simulink library "mach_lib"  (Simulink 6.3)
undefined symbols (not defined in the file): accel_cmd, aero_surf_qbar_off, aero_surf_qbar_on, altitude_stop, angular_rate_stop, att_cmd_select, att_trim_IC, att_type, att_type_numbers, bb_ellipsoid, bb_params, chi_trim_IC, command_time, compute_all_rate_cols, compute_all_vel_cols, constants, cosA, da_trim_IC, de_trim_IC, DiscIntNeverNeededParam, dr_trim_IC, dtsim, E_rwy, E_trim_IC, Ed_cmd, Ed_trim_IC, energy_stop, eow_boundary, full_surf_llim, full_surf_ulim, gain_var_struct, gam_cmd_descent, gam_cmd_preflare, gamdot_cmd_descent, gamdot_cmd_flare, gamdot_cmd_preflare, gamma_trim_IC, h_trim_IC, hd_cmd, hd_trim_IC, ideal_vel_Kb, integrate_start_time_sim, integrate_state_sim, llim, MACH, MACH_att_fb, MACH_gain_mat, MACH_mass_IC, MACH_pos_IC, MACH_pqr_Bmat_IC, MACH_pqr_IC, MACH_pqr_u_IC, MACH_quat_IC, MACH_throttle_IC, MACH_U_nom_IC, MACH_vel_Bmat_IC, MACH_vel_cvdnom_IC, MACH_vel_IC, MACH_vel_uold_IC, max_chi_cmd ... (+67)
libraries: simulink x75, mach_lib x27, utility_lib x25, model_lib x7, models x6
(part 3 of 6)

== system mach_lib/claw_main/input processing/set control parameters ==
  note: (Optionally) disable bb
      |  while we still have fuel
  signal_bus : Inport
  full_surf : Inport  Port=2
  Bus Creator1 : BusCreator  Inputs=10
  Bus Selector1 : BusSelector  OutputSignals=mode_sw.enable_bb_sw,mode_sw.gain_set_sw
  Bus Selector3 : BusSelector  OutputSignals=aero_env_est
  Constant : Constant
  Constant1 : Constant
  Logical Operator : Logic  Operator=NOT  AllPortsSameDT=off
  Logical Operator1 : Logic  Operator=NOT  AllPortsSameDT=off
  Logical Operator4 : Logic  AllPortsSameDT=off
  Logical Operator5 : Logic  Operator=OR  AllPortsSameDT=off
  accel submode setup : Subsystem
  modify MACH_att_Kf : Subsystem
  out of fuel : model_lib/out of fuel ?
  select gains : Subsystem
  set att desdyn params : Subsystem
  set pos desdyn params : Subsystem
  set rate desdyn params : Subsystem
  set rate di params : Subsystem
  set vel desdyn params : Subsystem
  control_params : Outport
  wires:
  modify MACH_att_Kf/1(gain_bus) -> set att desdyn params/1(gain_bus)
  full_surf/1 -> set rate di params/1(full_surf)
  Bus Selector3/1 -> set rate di params/2(aero_env_est)  "<aero_env_est>"
  set rate di params/1(rate_params) -> Bus Creator1/10  "rate_params"
  signal_bus/1 -> modify MACH_att_Kf/2(signal_bus), Bus Selector3/1, Bus Selector1/1, accel submode setup/1(signal_bus)
  accel submode setup/1(accel_cmd_sw) -> Bus Creator1/1  "accel_cmd_sw"
  accel submode setup/2(accel_cmd) -> Bus Creator1/2  "accel_cmd"
  Bus Selector1/2 -> select gains/2(gain_set_in)  "<gain_set_sw>"
  Constant1/1 -> Logical Operator5/2
  Logical Operator5/1 -> Logical Operator4/2
  Logical Operator1/1 -> Logical Operator5/1
  out of fuel/1 -> Logical Operator1/1
  Constant/1 -> out of fuel/1
  select gains/1(gain_set) -> Bus Creator1/5  "gain_set"
  Bus Creator1/1 -> control_params/1
  select gains/2(gain_bus) -> modify MACH_att_Kf/1(gain_bus_in), set rate desdyn params/1(gain_bus), set vel desdyn params/1(gain_bus), set pos desdyn params/1(gain_bus)
  Logical Operator4/1 -> Bus Creator1/4, Logical Operator/1, select gains/1(enable_bb)  "enable_bb"
  Logical Operator/1 -> Bus Creator1/3  "limit_pqr_cmd"
  Bus Selector1/1 -> Logical Operator4/1  "<enable_bb_sw>"
  set rate desdyn params/1(params) -> Bus Creator1/9  "rate_desdyn"
  set att desdyn params/1(params) -> Bus Creator1/8  "att_desdyn"
  set vel desdyn params/1(params) -> Bus Creator1/7  "vel_desdyn"
  set pos desdyn params/1(params) -> Bus Creator1/6  "pos_desdyn"

== system mach_lib/claw_main/pos_loops/compute trim ==
  inner cmd : Inport
  cmd : Inport  Port=2
  Sum1 : Sum  Inputs=|+-  SaturateOnIntegerOverflow=on
  trim : Outport
  wires:
  cmd/1 -> Sum1/2
  inner cmd/1 -> Sum1/1
  Sum1/1 -> trim/1

== system mach_lib/claw_main/pos_loops/limiter ==
  vel_inner_cmd : Inport
  signal_bus : Inport  Port=2
  cvd_des_in : Inport  Port=3
  Bus Selector2 : BusSelector  OutputSignals=cmd_bus.select_cmd.vel,feed_forward.pos_ff,y_meas.dc_fltpath
  Compare To Constant : simulink/Logic and Bit Operations/Compare To Constant  relop=<  const=2  LogicOutDataTypeMode=boolean  ZeroCross=off
  Constant : Constant  Value=use_pos_fltpath_lim
  Math Function : Math  Operator=transpose  SaturateOnIntegerOverflow=on
  Product : Product  Multiplication=Matrix(*)  RndMeth=Zero
  Product1 : Product  Multiplication=Matrix(*)  RndMeth=Zero
  Saturation : Saturate  UpperLimit=MACH.pos_u_ulim  LowerLimit=MACH.pos_u_llim
  Saturation1 : Saturate  UpperLimit=MACH.pos_fltpath_u_ulim  LowerLimit=MACH.pos_fltpath_u_llim
  Selector1 : Selector  Elements=[1 2 4]  InputPortWidth=4
  Sum : Sum  Inputs=-+|
  Sum1 : Sum  Inputs=++|
  Sum2 : Sum  Inputs=+-|  SaturateOnIntegerOverflow=on  InputSameDT=on
  Switch : Switch  Threshold=0.5
  Switch1 : Switch  Threshold=0.5
  Unit Delay : UnitDelay  X0=MACH_vel_IC  SampleTime=MACH.dt
  cvd_des : Outport
  cvd_extra : Outport  Port=2
  wires:
  vel_inner_cmd/1 -> Unit Delay/1
  Unit Delay/1 -> Switch1/1
  Selector1/1 -> Compare To Constant/1
  Compare To Constant/1 -> Switch1/2
  Bus Selector2/2 -> Switch1/3  "<pos_ff>"
  Bus Selector2/1 -> Selector1/1  "<vel>"
  signal_bus/1 -> Bus Selector2/1
  Sum2/1 -> cvd_extra/1
  Product1/1 -> Sum1/2
  Math Function/1 -> Product1/1
  Saturation1/1 -> Product1/2
  Product/1 -> Saturation1/1
  Sum/1 -> Product/2
  Bus Selector2/3 -> Math Function/1, Product/1  "<dc_fltpath>"
  cvd_des_in/1 -> Sum2/2, Saturation/1, Sum/2
  Sum1/1 -> Switch/1
  Switch/1 -> Sum2/1, cvd_des/1
  Saturation/1 -> Switch/3
  Constant/1 -> Switch/2
  Switch1/1 -> Sum/1, Sum1/1

== system mach_lib/claw_main/pos_loops/select pos cmd ==
  NEh_current : Inport
  outer cmd : Inport  Port=2
  signal_bus : Inport  Port=3
  Bus Selector : BusSelector  OutputSignals=cmd_bus.select_cmd.pos,cmd_bus.autopilot_cmd
  Demux3 : Demux  Outputs=[ 3 1 ]
  Ground : Ground
  Multiport Switch : MultiPortSwitch  Inputs=3  zeroidx=on  SaturateOnIntegerOverflow=on
  Mux1 : Mux  Inputs=2
  Selector2 : Selector  Elements=[1 2 4 3]  InputPortWidth=4
  Selector4 : Selector  Elements=[1 2 4 3]  InputPortWidth=4
  NEh_cmd : Outport
  cam_cmd : Outport  Port=2
  cmd : Outport  Port=3
  wires:
  signal_bus/1 -> Bus Selector/1
  Demux3/2 -> cam_cmd/1
  Demux3/1 -> NEh_cmd/1
  Selector4/1 -> Demux3/1
  Selector2/1 -> Multiport Switch/2
  Mux1/1 -> Selector2/1
  Ground/1 -> Mux1/2
  NEh_current/1 -> Mux1/1
  Bus Selector/1 -> Multiport Switch/1  "<pos>"
  Bus Selector/2 -> Multiport Switch/3  "<autopilot_cmd>"
  outer cmd/1 -> Multiport Switch/4
  Multiport Switch/1 -> Selector4/1, cmd/1

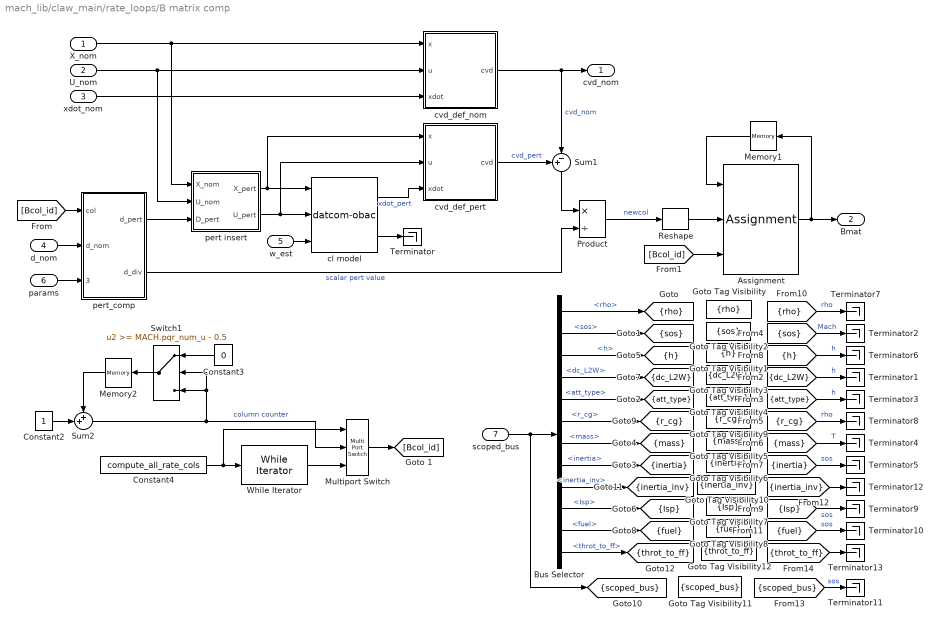
== system mach_lib/claw_main/rate_loops/B matrix comp ==
  X_nom : Inport
  U_nom : Inport  Port=2
  xdot_nom : Inport  Port=3
  d_nom : Inport  Port=4
  w_est : Inport  Port=5
  params : Inport  Port=6
  scoped_bus : Inport  Port=7
  Assignment : Assignment  InputType=Matrix  Rows=-1  ColumnSrc=External
  Bus Selector : BusSelector  OutputSignals=atmos_env.rho,atmos_env.sos,atmos_env.h,dc_L2W,att_type,mass_props.r_cg,mass_props.mass,mass_props.inertia,mass_props.inertia_inv,mass_props.Isp,mass_props.fuel,mass_props.throt_to_ff
  Constant2 : Constant
  Constant3 : Constant  Orientation=left  Value=0
  Constant4 : Constant  Value=compute_all_rate_cols
  Goto Tag Visibility : GotoTagVisibility  GotoTag=rho
  Goto Tag Visibility1 : GotoTagVisibility  GotoTag=h
  Goto Tag Visibility10 : GotoTagVisibility  GotoTag=inertia_inv
  Goto Tag Visibility11 : GotoTagVisibility  GotoTag=scoped_bus
  Goto Tag Visibility12 : GotoTagVisibility  GotoTag=throt_to_ff
  Goto Tag Visibility2 : GotoTagVisibility  GotoTag=sos
  Goto Tag Visibility3 : GotoTagVisibility  GotoTag=dc_L2W
  Goto Tag Visibility4 : GotoTagVisibility  GotoTag=att_type
  Goto Tag Visibility5 : GotoTagVisibility  GotoTag=mass
  Goto Tag Visibility6 : GotoTagVisibility  GotoTag=inertia
  Goto Tag Visibility7 : GotoTagVisibility  GotoTag=Isp
  Goto Tag Visibility8 : GotoTagVisibility  GotoTag=fuel
  Goto Tag Visibility9 : GotoTagVisibility  GotoTag=r_cg
  Memory1 : Memory  Orientation=left  X0=MACH_pqr_Bmat_IC  InheritSampleTime=on
  Memory2 : Memory  Orientation=left  InheritSampleTime=on
  Multiport Switch : MultiPortSwitch  Inputs=2  zeroidx=on
  Product : Product  Inputs=*/  SaturateOnIntegerOverflow=on  InputSameDT=on
  Reshape : simulink/Math Operations/Reshape  OutputDimensionality=Column vector  OutputDimensions=[1,1]
  Sum1 : Sum  Orientation=down  Inputs=+-|  SaturateOnIntegerOverflow=on  InputSameDT=on
  Sum2 : Sum  Inputs=++|  SaturateOnIntegerOverflow=on  InputSameDT=on
  Switch1 : Switch  Orientation=left  Threshold=MACH.pqr_num_u - 0.5  SaturateOnIntegerOverflow=on  InputSameDT=on
  Terminator{,1..13} (14 alike) : Terminator
  While Iterator : WhileIterator  MaxIters=MACH.pqr_num_u  WhileBlockType=do-while  ShowIterationPort=on
  cl model : models/datcom-obac
  cvd_def_nom : Subsystem
  cvd_def_pert : Subsystem
  pert insert : Subsystem
  pert_comp : Subsystem
  cvd_nom : Outport
  Bmat : Outport  Port=2
  tag scope: Isp=scoped, att_type=scoped, dc_L2W=scoped, fuel=scoped, h=scoped, inertia=scoped, inertia_inv=scoped, mass=scoped, r_cg=scoped, rho=scoped, scoped_bus=scoped, sos=scoped, throt_to_ff=scoped
  wires:
  Bus Selector/12 -> [throt_to_ff]  "<throt_to_ff>"
  [throt_to_ff] -> Terminator13/1
  [scoped_bus] -> Terminator11/1  "sos"
  Bus Selector/9 -> [inertia_inv]  "<inertia_inv>"
  [inertia_inv] -> Terminator12/1
  Bus Selector/11 -> [fuel]  "<fuel>"
  [fuel] -> Terminator10/1  "sos"
  Bus Selector/10 -> [Isp]  "<Isp>"
  [Isp] -> Terminator9/1  "sos"
  Bus Selector/8 -> [inertia]  "<inertia>"
  Bus Selector/7 -> [mass]  "<mass>"
  Bus Selector/6 -> [r_cg]  "<r_cg>"
  [inertia] -> Terminator5/1  "sos"
  [mass] -> Terminator4/1  "T"
  [r_cg] -> Terminator8/1  "rho"
  Bus Selector/5 -> [att_type]  "<att_type>"
  [att_type] -> Terminator3/1  "h"
  Bus Selector/4 -> [dc_L2W]  "<dc_L2W>"
  [dc_L2W] -> Terminator1/1  "h"
  Bus Selector/3 -> [h]  "<h>"
  Bus Selector/2 -> [sos]  "<sos>"
  Bus Selector/1 -> [rho]  "<rho>"
  [h] -> Terminator6/1  "h"
  [sos] -> Terminator2/1  "Mach"
  [rho] -> Terminator7/1  "rho"
  scoped_bus/1 -> [scoped_bus], Bus Selector/1
  Multiport Switch/1 -> [Bcol_id]
  Constant2/1 -> Sum2/2
  Memory2/1 -> Sum2/1
  Switch1/1 -> Memory2/1
  Sum2/1 -> Multiport Switch/2, Switch1/2, Switch1/3  "column counter"
  Constant3/1 -> Switch1/1
  While Iterator/1 -> Multiport Switch/3
  Constant4/1 -> While Iterator/1, Multiport Switch/1
  params/1 -> pert_comp/3(params)
  cl model/2 -> Terminator/1
  Memory1/1 -> Assignment/1
  d_nom/1 -> pert_comp/2(d_nom)
  w_est/1 -> cl model/3
  cl model/1 -> cvd_def_pert/3(xdot)  "xdot_pert"
  cvd_def_nom/1(cvd) -> cvd_nom/1, Sum1/2  "cvd_nom"
  cvd_def_pert/1(cvd) -> Sum1/1  "cvd_pert"
  xdot_nom/1 -> cvd_def_nom/3(xdot)
  U_nom/1 -> pert insert/2(U_nom), cvd_def_nom/2(u)
  X_nom/1 -> pert insert/1(X_nom), cvd_def_nom/1(x)
  Product/1 -> Reshape/1  "newcol"
  Sum1/1 -> Product/1
  [Bcol_id] -> Assignment/3
  Assignment/1 -> Memory1/1, Bmat/1
  [Bcol_id] -> pert_comp/1(col)
  pert_comp/2(d_div) -> Product/2  "scalar pert value"
  pert insert/2(U_pert) -> cl model/2, cvd_def_pert/2(u)
  pert insert/1(X_pert) -> cl model/1, cvd_def_pert/1(x)
  pert_comp/1(d_pert) -> pert insert/3(D_pert)
  Reshape/1 -> Assignment/2

== system mach_lib/claw_main/rate_loops/allocation ==
  cvd_nom : Inport
  Bmat : Inport  Port=2
  d_old : Inport  Port=3
  d_nom : Inport  Port=4
  cvd_des : Inport  Port=5
  params : Inport  Port=6
  Bmat_rcs : Selector  InputType=Matrix  Elements=MACH.pqr_u_idx  Rows=-1  Columns=MACH.pqr_u_rcs_idx  InputPortWidth=MACH.num_u
  Bmat_smn : Selector  InputType=Matrix  Elements=MACH.pqr_u_idx  Rows=-1  Columns=MACH.pqr_u_smn_idx  InputPortWidth=MACH.num_u
  Gain : Gain  Gain=-1
  Mux3 : Mux  Inputs=2
  RCS allocation : Subsystem
  Selector : Selector  InputType=Matrix  Elements=MACH.pqr_u_idx  Rows=1:9  Columns=1:2  InputPortWidth=MACH.num_u
  config_di : Subsystem  BlockChoice=di_smn  mask{num_cv=MACH.pqr_num_cv, num_u=MACH.pqr_num_u_smn, wght_cv_type=MACH.pqr_wght_cv_type}
      link override di_smn/config_smn/smn_sfunc: sfunc_name=MACH.smn_sfunc_name
      settings: AttributesFormatString=%<BlockChoice>  TemplateBlock=mach_lib/config_di  MemberBlocks=di_pseudoinv,di_smn
  d_nom_smn : Selector  Elements=MACH.pqr_u_smn_idx  InputPortWidth=MACH.pqr_num_u
  d_old_rcs : Selector  Elements=MACH.pqr_u_rcs_idx  InputPortWidth=MACH.pqr_num_u
  d_old_smn : Selector  Elements=MACH.pqr_u_smn_idx  InputPortWidth=MACH.pqr_num_u
  param select rcs : Subsystem  mask{idx=MACH.pqr_u_rcs_idx}
      mask prompts: idx "index"
  param select smn : Subsystem  mask{idx=MACH.pqr_u_smn_idx}
      mask prompts: idx "index"
  d_cmd : Outport
  cvd_extra_smn : Outport  Port=2
  lambda : Outport  Port=3
  solve_dat : Outport  Port=4
  cvd_extra : Outport  Port=5
  wires:
  param select rcs/1(params) -> RCS allocation/4(params)
  params/1 -> param select rcs/1(params_all), param select smn/1(params_all)
  Selector/1 -> solve_dat/1
  param select smn/1(params) -> config_di/6(params)
  RCS allocation/2(cvd_extra) -> cvd_extra/1
  cvd_des/1 -> config_di/5(cvd_des)
  config_di/3(lambda) -> lambda/1
  d_old/1 -> [d_old], d_old_smn/1
  Mux3/1 -> d_cmd/1
  d_nom/1 -> d_nom_smn/1
  Bmat/1 -> [Bmat], Bmat_smn/1
  cvd_nom/1 -> config_di/1(cvd_nom)
  config_di/4(solve_dat) -> Selector/1
  config_di/2(cvd_extra) -> cvd_extra_smn/1, Gain/1  "cvdex_smn"
  [d_old] -> d_old_rcs/1
  Gain/1 -> RCS allocation/3(cvd_des)
  Bmat_smn/1 -> config_di/2(Bmat)
  d_old_rcs/1 -> RCS allocation/2(rcs_cmd_old)
  RCS allocation/1(rcs_cmd) -> Mux3/2
  [Bmat] -> Bmat_rcs/1
  Bmat_rcs/1 -> RCS allocation/1(Bmat)
  d_old_smn/1 -> config_di/3(d_old)
  d_nom_smn/1 -> config_di/4(d_nom)
  config_di/1(d_cmd) -> Mux3/1

== system mach_lib/claw_main/rate_loops/bangbang ==
  enable_bb : Inport
  att_cvc : Inport  Port=2
  att_cv : Inport  Port=3
  pqr : Inport  Port=4
  cvd_des_lin : Inport  Port=5
  Bang Bang : Stateflow chart
  Constant1 : Constant  Value=bb_params
  Constant2 : Constant  Value=bb_ellipsoid
  Mux : Mux  Inputs=[12 3 3 1 1 3]
  Unit Delay : UnitDelay  X0=[ 0 0 0 ]  SampleTime=MACH.dt
  Unit Delay1 : UnitDelay  SampleTime=MACH.dt
  Unit Delay2 : UnitDelay  SampleTime=MACH.dt
  cvd_des : Outport
  bb_debug : Outport  Port=2
  wires:
  Bang Bang/2(cvddes) -> Mux/2, cvd_des/1  "cvd_des"
  Mux/1 -> bb_debug/1
  Bang Bang/1(debug_output) -> Mux/1
  Constant2/1 -> Bang Bang/2(bb_ellipsoid)
  cvd_des_lin/1 -> Mux/6, Bang Bang/8(cvddes_lin)  "cvd_des_lin"
  Bang Bang/4(use_bb) -> Mux/4, Unit Delay2/1
  Unit Delay2/1 -> Bang Bang/10(use_bb_old)
  enable_bb/1 -> Bang Bang/7(enable_bb)
  [inertia] -> Bang Bang/6(inertia)
  Constant1/1 -> Bang Bang/1(bb_params)
  Unit Delay/1 -> Bang Bang/9(dir_old)
  Bang Bang/3(dir) -> Mux/3, Unit Delay/1
  Bang Bang/5(timer) -> Mux/5, Unit Delay1/1
  Unit Delay1/1 -> Bang Bang/11(timer_old)
  att_cv/1 -> Bang Bang/4(att_cv)
  pqr/1 -> Bang Bang/5(pqr)
  att_cvc/1 -> Bang Bang/3(att_cvc)

== system mach_lib/claw_main/rate_loops/compute trim ==
  inner cmd : Inport
  Bmat : Inport  Port=2
  cmd : Inport  Port=3
  Product : Product  Multiplication=Matrix(*)  SaturateOnIntegerOverflow=on
  Sum1 : Sum  Inputs=|+-  SaturateOnIntegerOverflow=on
  trim : Outport
  wires:
  cmd/1 -> Sum1/2
  inner cmd/1 -> Sum1/1
  Sum1/1 -> Product/2
  Bmat/1 -> Product/1
  Product/1 -> trim/1

== system mach_lib/claw_main/rate_loops/select rate cmd ==
  pqr_current : Inport
  throt_current : Inport  Port=2
  outer cmd : Inport  Port=3
  signal_bus : Inport  Port=4
  Bus Selector6 : BusSelector  OutputSignals=cmd_bus.select_cmd.rate
  Demux : Demux  Outputs=[ MACH.pqr_num_cv MACH.num_u_throt ]
  Multiport Switch : MultiPortSwitch  Inputs=3  zeroidx=on  SaturateOnIntegerOverflow=on
  Mux1 : Mux  Inputs=2
  Unit Delay1 : UnitDelay  X0=MACH_throttle_IC  SampleTime=-1
  get direct cmd : Subsystem
  select multiple throts : Selector  Elements=[1:3 4*ones(1,MACH.num_u_throt)]  InputPortWidth=4
  pqr_cmd : Outport
  throt_cmd : Outport  Port=2
  cmd : Outport  Port=3
  wires:
  Demux/2 -> throt_cmd/1
  Demux/1 -> pqr_cmd/1
  Bus Selector6/1 -> select multiple throts/1  "<rate>"
  signal_bus/1 -> Bus Selector6/1, get direct cmd/1(signal_bus)
  get direct cmd/1(direct_cmd) -> Multiport Switch/3
  throt_current/1 -> Unit Delay1/1
  pqr_current/1 -> Mux1/1
  Unit Delay1/1 -> Mux1/2
  select multiple throts/1 -> Multiport Switch/1
  Mux1/1 -> Multiport Switch/2
  outer cmd/1 -> Multiport Switch/4
  Multiport Switch/1 -> Demux/1, cmd/1

== system mach_lib/claw_main/rate_loops/set rate loop params ==
  rate_params : Inport
  u_old : Inport  Port=2
  Bus Assignment : BusAssignment  AssignedSignals=u_ulim,u_llim
  Bus Selector1 : BusSelector  OutputSignals=u_ulim,u_llim,u_urlim,u_lrlim
  rate limit limits : mach_lib/rate limit limits  ulim=MACH.pqr_u_ulim  llim=MACH.pqr_u_llim
  params : Outport
  wires:
  Bus Assignment/1 -> params/1
  rate limit limits/2 -> Bus Assignment/3
  rate limit limits/1 -> Bus Assignment/2
  Bus Selector1/4 -> rate limit limits/5  "<u_lrlim>"
  Bus Selector1/3 -> rate limit limits/4  "<u_urlim>"
  Bus Selector1/2 -> rate limit limits/3  "<u_llim>"
  Bus Selector1/1 -> rate limit limits/2  "<u_ulim>"
  rate_params/1 -> Bus Assignment/1, Bus Selector1/1
  u_old/1 -> rate limit limits/1

== system mach_lib/claw_main/servo commands  when not engaged/pseudo surf cmd ==
  autopilot_cmd : Inport
  Assignment1 : Assignment  Elements=[ MACH.vane_idx MACH.throttle_idx ]  OutputInitialize=Initialize using input (U1)
  Constant : Constant  Value=MACH_U_nom_IC
  Demux2 : Demux  Outputs=[ 3 1 ]
  Gain : Gain  Gain=MACH.mixer  Multiplication=Matrix(K*u)  SaturateOnIntegerOverflow=on
  Gain1 : Gain  Gain=MACH.throt_mixer
  Mux : Mux  Inputs=2
  surf_cmd : Outport
  wires:
  Constant/1 -> Assignment1/1
  Assignment1/1 -> surf_cmd/1
  autopilot_cmd/1 -> Demux2/1
  Demux2/1 -> Gain/1  "da,de,dr"
  Demux2/2 -> Gain1/1  "throttle"
  Gain/1 -> Mux/1
  Gain1/1 -> Mux/2
  Mux/1 -> Assignment1/2

== system mach_lib/claw_main/state est/process inputs ==
  u_old : Inport
  sensors : Inport  Port=2
  Bus Selector2 : BusSelector  OutputSignals=u_meas
  Constant : Constant  Value=0
  Multiport Switch1 : MultiPortSwitch  Inputs=2  zeroidx=on  SaturateOnIntegerOverflow=on
  throt : Selector  Elements=MACH.throttle_idx  InputPortWidth=MACH.num_u
  use throt estimate from measurement instead of past throt cmd : Assignment  Elements=MACH.throttle_idx
  use_throt_estimate : Constant  Value=use_throt_estimate
  zero RCS inputs : Assignment  Elements=MACH.rcs_idx  OutputInitialize=Initialize using input (U1)
  u_est : Outport
  wires:
  throt/1 -> use throt estimate from measurement instead of past throt cmd/2
  zero RCS inputs/1 -> u_est/1
  Constant/1 -> zero RCS inputs/2
  Multiport Switch1/1 -> zero RCS inputs/1
  Bus Selector2/1 -> throt/1  "<u_meas>"
  sensors/1 -> Bus Selector2/1
  use throt estimate from measurement instead of past throt cmd/1 -> Multiport Switch1/3
  use_throt_estimate/1 -> Multiport Switch1/1
  u_old/1 -> Multiport Switch1/2, use throt estimate from measurement instead of past throt cmd/1

== system mach_lib/claw_main/state est/process sensors ==
  reset_pos : Inport
  nav_ok : Inport  Port=2
  pqr : Inport  Port=3
  NED_dot : Inport  Port=4
  latlonh : Inport  Port=5
  e : Inport  Port=6
  Bus Creator : BusCreator
  Gain : Gain  Gain=[1 1 -1]  SaturateOnIntegerOverflow=on
  Gain1 : Gain  Gain=[1 1 0]  SaturateOnIntegerOverflow=on
  LLh2NEh : utility_lib/LLh2NEh
  Product : Product  Multiplication=Matrix(*)  SaturateOnIntegerOverflow=on
  Reshape : simulink/Math Operations/Reshape  OutputDimensionality=Customize  OutputDimensions=[3,3]
  Selector : Selector  Elements=[3]  InputPortWidth=3
  Sum : Sum  Inputs=|+-  SaturateOnIntegerOverflow=on
  Switch1 : Switch  Threshold=0.5  SaturateOnIntegerOverflow=on
  Switch2 : Switch  Threshold=0.5  SaturateOnIntegerOverflow=on
  Unit Delay : UnitDelay  Orientation=left  SampleTime=-1
  Unit Delay1 : UnitDelay  Orientation=left  X0=MACH_quat_IC  SampleTime=-1
  compute dc_fltpath : Subsystem
  e2dc : utility_lib/e2dc
  navigation complementary filter : Subsystem
  select e sign : Subsystem
  use_nav : Constant  Value=use_nav
  wait for valid nav : Subsystem
  vehicle_origin : Outport
  h_geodetic : Outport  Port=2
  NEh_nav : Outport  Port=3
  nav_valid : Outport  Port=4
  NEh_dot : Outport  Port=5
  dc_fltpath : Outport  Port=6
  cvc_origin : Outport  Port=7
  dircos : Outport  Port=8
  x_est : Outport  Port=9
  wires:
  compute dc_fltpath/1(dc_fltpath) -> dc_fltpath/1
  Gain1/1 -> vehicle_origin/1, LLh2NEh/2
  Selector/1 -> h_geodetic/1
  Bus Creator/1 -> x_est/1
  Product/1 -> Bus Creator/2  "uvw"
  pqr/1 -> Bus Creator/1  "pqr"
  Reshape/1 -> Product/1
  select e sign/1(e out) -> Bus Creator/4, e2dc/1, Unit Delay1/1  "e"
  Gain/1 -> NEh_dot/1, compute dc_fltpath/1(NEh_dot_fltpath), navigation complementary filter/2(NEh dot)
  NED_dot/1 -> Gain/1, Product/2
  e2dc/1 -> Reshape/1, dircos/1
  latlonh/1 -> Selector/1, LLh2NEh/1, wait for valid nav/1(latlonh)
  reset_pos/1 -> Switch1/2
  nav_ok/1 -> wait for valid nav/2(nav_ok)
  wait for valid nav/2(nav_valid) -> nav_valid/1
  LLh2NEh/1 -> Switch2/1, navigation complementary filter/1(NEh nav)
  Switch1/1 -> Sum/2, cvc_origin/1, Unit Delay/1  "NEh"
  Unit Delay/1 -> Switch1/3
  Switch2/1 -> Switch1/1, NEh_nav/1, Sum/1
  use_nav/1 -> Switch2/2
  navigation complementary filter/1(NEh_fil) -> Switch2/3
  Sum/1 -> Bus Creator/3  "NEh"
  wait for valid nav/1(LLh_0) -> Gain1/1
  Unit Delay1/1 -> select e sign/2(e_past)
  e/1 -> select e sign/1(e in)

== system mach_lib/claw_main/state est/wind estimator ==
  dircos : Inport
  x : Inport  Port=2
  sensors : Inport  Port=3
  u : Inport  Port=4
  wind_est_sw : Inport  Port=5
  Bus Selector1 : BusSelector  OutputSignals=NED_wind,accels_cg
  Bus Selector2 : BusSelector  OutputSignals=accels_cg
  Multiport Switch1 : MultiPortSwitch  Inputs=2  zeroidx=on  SaturateOnIntegerOverflow=on
  Unit Delay : UnitDelay  X0=zeros(3,1)  SampleTime=-1
  cl model : models/datcom-obac
  use_wind_est : Constant  Value=use_wind_est
  wind estimate : Subsystem
  w_est : Outport
  w_est_debug : Outport  Port=2
  wires:
  Bus Selector2/1 -> wind estimate/4(model_accels_cg)  "<accels_cg>"
  cl model/2 -> Bus Selector2/1
  Bus Selector1/2 -> wind estimate/5(sensed_accels_cg)  "<accels_cg>"
  Bus Selector1/1 -> Multiport Switch1/2  "<NED_wind>"
  wind estimate/2(w_est_debug) -> w_est_debug/1
  sensors/1 -> Bus Selector1/1
  wind_est_sw/1 -> wind estimate/6(wind_est_sw)
  Multiport Switch1/1 -> w_est/1
  dircos/1 -> wind estimate/1(dircos)
  u/1 -> cl model/2
  x/1 -> cl model/1, wind estimate/2(x)
  wind estimate/1(w_est) -> Multiport Switch1/3, Unit Delay/1
  use_wind_est/1 -> Multiport Switch1/1
  Unit Delay/1 -> cl model/3
  cl model/1 -> wind estimate/3(xdot)

== system mach_lib/claw_main/vel_loops/B matrix comp ==
  note: Note: Ideally,  X_nom and U_nom
      |  would be constructed to be near
      |  moment equalibrium
  X : Inport
  U_limited : Inport  Port=2
  d_nom : Inport  Port=3
  camcmd : Inport  Port=4
  params : Inport  Port=5
  w_est : Inport  Port=6
  NEh_dot : Inport  Port=7
  scoped_bus : Inport  Port=8
  B matrix comp : Subsystem  TreatAsAtomicUnit=on
  Constant : Constant  Value=0
  Constant1 : Constant  Value=0
  compute cvd_nom : Subsystem
  compute nominal XU : Subsystem
  zero pqr : Assignment  Elements=MACH.pqr_idx  OutputInitialize=Initialize using input (U1)
  zero rate surfs : Assignment  Elements=MACH.pqr_u_idx  OutputInitialize=Initialize using input (U1)
  cvd_nom : Outport
  Bmat : Outport  Port=2
  wires:
  X/1 -> zero pqr/1
  U_limited/1 -> zero rate surfs/1
  Constant1/1 -> zero rate surfs/2
  Constant/1 -> zero pqr/2
  zero pqr/1 -> compute nominal XU/1(X_in)
  zero rate surfs/1 -> compute nominal XU/2(U_in)
  compute nominal XU/2(U_out) -> B matrix comp/3(U_nom), compute cvd_nom/2(u)
  compute nominal XU/1(X_out) -> B matrix comp/2(X_nom), compute cvd_nom/1(x)
  B matrix comp/1(Bmat) -> Bmat/1
  w_est/1 -> compute cvd_nom/3(w_est), B matrix comp/4(w_est)
  compute cvd_nom/1(cvd) -> B matrix comp/1(cvd_nom), cvd_nom/1
  NEh_dot/1 -> compute nominal XU/5(NEh_dot), B matrix comp/7(NEh_dot)
  params/1 -> B matrix comp/8(params)
  d_nom/1 -> compute nominal XU/3(D_in), B matrix comp/5(d_nom)
  scoped_bus/1 -> B matrix comp/9(scoped_bus)
  camcmd/1 -> compute nominal XU/4(camcmd), B matrix comp/6(camcmd)

== system mach_lib/claw_main/vel_loops/compute trim ==
  inner cmd : Inport
  Bmat : Inport  Port=2
  cmd : Inport  Port=3
  Product : Product  Multiplication=Matrix(*)  SaturateOnIntegerOverflow=on
  Sum1 : Sum  Inputs=|+-  SaturateOnIntegerOverflow=on
  trim : Outport
  wires:
  cmd/1 -> Sum1/2
  inner cmd/1 -> Sum1/1
  Sum1/1 -> Product/2
  Bmat/1 -> Product/1
  Product/1 -> trim/1

== system mach_lib/claw_main/vel_loops/config_di ==
  cvd_nom : Inport
  Bmat : Inport  Port=2
  d_old : Inport  Port=3
  d_nom : Inport  Port=4
  cvd_des : Inport  Port=5
  params : Inport  Port=6
  di_smn : mach_lib/di_smn
  d_cmd : Outport
  cvd_extra : Outport  Port=2
  lambda : Outport  Port=3
  solve_dat : Outport  Port=4
  wires:
  di_smn/4 -> solve_dat/1
  di_smn/3 -> lambda/1
  di_smn/2 -> cvd_extra/1
  di_smn/1 -> d_cmd/1
  params/1 -> di_smn/6
  cvd_des/1 -> di_smn/5
  d_nom/1 -> di_smn/4
  d_old/1 -> di_smn/3
  Bmat/1 -> di_smn/2
  cvd_nom/1 -> di_smn/1

== system mach_lib/claw_main/vel_loops/convert accel_cmd to NED_dd_cmd ==
  accel_cmd : Inport
  accel_cmd_sw : Inport  Port=2
  NEh_d : Inport  Port=3
  Merge : Merge  InitialOutput=zeros(3,1)
  MinMax : MinMax  Function=max
  NED_dd cmd : Subsystem  TreatAsAtomicUnit=on
  Switch Case : SwitchCase  CaseConditions={1,2}  CaseShowDefault=off
  vchigam_dot cmd : Subsystem  TreatAsAtomicUnit=on
  NEh_dd_cmd : Outport
  wires:
  NED_dd cmd/1(NEh_dd_cmd) -> Merge/1
  accel_cmd/1 -> NED_dd cmd/1(NEH_dd_cmd_in), vchigam_dot cmd/1(vchigam_dot_cmd)
  Switch Case/2 -> vchigam_dot cmd/Action
  Switch Case/1 -> NED_dd cmd/Action
  Merge/1 -> NEh_dd_cmd/1
  vchigam_dot cmd/1(NEh_dd_cmd) -> Merge/2
  NEh_d/1 -> vchigam_dot cmd/2(NEh_d)
  MinMax/1 -> Switch Case/1
  accel_cmd_sw/1 -> MinMax/1

== system mach_lib/claw_main/vel_loops/from inner ==
  att,T : Inport
  Demux1 : Demux  Outputs=[ 2 1 MACH.num_u_throt ]
  Mux1 : Mux  Inputs=2
  Terminator : Terminator
  d_cmd : Outport
  wires:
  Demux1/2 -> Terminator/1
  Demux1/3 -> Mux1/2
  Mux1/1 -> d_cmd/1
  Demux1/1 -> Mux1/1
  att,T/1 -> Demux1/1

== system mach_lib/claw_main/vel_loops/from quat ==
  e,T : Inport
  Demux1 : Demux  Outputs=[ 4 MACH.num_u_throt ]
  Mux1 : Mux  Inputs=2
  Selector1 : Selector  Elements=1:2  InputPortWidth=3
  e2att : utility_lib/e2att
  d_cmd : Outport
  wires:
  e,T/1 -> Demux1/1
  Demux1/1 -> e2att/1
  Mux1/1 -> d_cmd/1
  Demux1/2 -> Mux1/2
  Selector1/1 -> Mux1/1
  e2att/1 -> Selector1/1

== system mach_lib/claw_main/vel_loops/select vel cmd ==
  NEh_dot_current : Inport
  cam_current : Inport  Port=2
  outer cmd : Inport  Port=3
  signal_bus : Inport  Port=4
  Bus Selector : BusSelector  OutputSignals=cmd_bus.select_cmd.vel,cmd_bus.autopilot_cmd
  Demux3 : Demux  Outputs=[ MACH.vel_num_cv 1 ]
  Multiport Switch : MultiPortSwitch  Inputs=3  zeroidx=on  SaturateOnIntegerOverflow=on
  Mux : Mux  Inputs=2
  Selector1 : Selector  Elements=[1 2 4 3]  InputPortWidth=4
  Selector2 : Selector  Elements=[1 2 4 3]  InputPortWidth=4
  NEh_dot_cmd : Outport
  cam_cmd : Outport  Port=2
  cmd : Outport  Port=3
  wires:
  cam_current/1 -> Mux/2
  Bus Selector/2 -> Multiport Switch/3  "<autopilot_cmd>"
  signal_bus/1 -> Bus Selector/1
  Selector1/1 -> Multiport Switch/2
  NEh_dot_current/1 -> Mux/1
  Mux/1 -> Selector1/1
  Demux3/2 -> cam_cmd/1
  Demux3/1 -> NEh_dot_cmd/1
  Selector2/1 -> Demux3/1
  Bus Selector/1 -> Multiport Switch/1  "<vel>"
  outer cmd/1 -> Multiport Switch/4
  Multiport Switch/1 -> Selector2/1, cmd/1

== system mach_lib/claw_main/vel_loops/set di params ==
  note: Note: dc_fltpath is now computed from NEh_dot.
      | Switch to recover old computation base on NEh_dot_cmd
  NEh_dot_cmd : Inport
  full_surf : Inport  Port=2
  u_old : Inport  Port=3
  uvw : Inport  Port=4
  dc_fltpath : Inport  Port=5
  Bus Creator1 : BusCreator  Inputs=7
  Bus Selector : BusSelector  OutputSignals=u_ulim,u_llim,u_urlim,u_lrlim
  Bus Selector1 : BusSelector  OutputSignals=throt_ulim,throt_llim
  Constant1 : Constant  Value=MACH.vel_wght_cv
  Constant3 : Constant  Value=MACH.vel_u_pref
  Constant4 : Constant  Value=MACH.vel_wght_u_pref
  Demux1 : Demux  Outputs=[ 2 MACH.num_u_throt ]
  Gain2 : Gain  Gain=repmat(MACH.vel_wght_fltpath',1,3)
  Logical Operator : Logic  Inputs=1  AllPortsSameDT=off  OutDataTypeMode=Boolean
  Manual Switch : simulink/Signal Routing/Manual Switch  sw=1  action=0
  Multiport Switch2 : MultiPortSwitch  Inputs=2  zeroidx=on
  Relational Operator : RelationalOperator  Operator===  LogicOutDataTypeMode=Boolean
  Terminator : Terminator
  att limits : Subsystem
  combine limits : Subsystem
  compute dc_fltpath : Subsystem
  throttle limits : Subsystem
  params : Outport
  wires:
  compute dc_fltpath/1(dc_fltpath) -> Manual Switch/2
  dc_fltpath/1 -> Manual Switch/1
  Manual Switch/1 -> Gain2/1
  NEh_dot_cmd/1 -> compute dc_fltpath/1(NEh_dot_fltpath)
  Gain2/1 -> Multiport Switch2/3
  u_old/1 -> Demux1/1
  Demux1/1 -> Terminator/1
  Demux1/2 -> throttle limits/2(throt_old)
  Bus Selector1/2 -> Relational Operator/2  "<throt_llim>"
  Bus Selector1/1 -> Relational Operator/1  "<throt_ulim>"
  Bus Selector/3 -> Bus Creator1/3  "<u_urlim>"
  combine limits/1(vel_u_limits) -> Bus Selector/1
  throttle limits/1(throt_limits) -> Bus Selector1/1, combine limits/2(throt_limits)
  att limits/1(att_limits) -> combine limits/1(att_limits)
  uvw/1 -> att limits/1(uvw)
  Logical Operator/1 -> Multiport Switch2/1
  Relational Operator/1 -> Logical Operator/1
  Bus Creator1/1 -> params/1
  Bus Selector/4 -> Bus Creator1/4  "<u_lrlim>"
  Bus Selector/2 -> Bus Creator1/2  "<u_llim>"
  Bus Selector/1 -> Bus Creator1/1  "<u_ulim>"
  full_surf/1 -> throttle limits/1(full_surf)
  Constant1/1 -> Multiport Switch2/2
  Multiport Switch2/1 -> Bus Creator1/7  "wght_cv"
  Constant3/1 -> Bus Creator1/5  "u_pref"
  Constant4/1 -> Bus Creator1/6  "wght_u_pref"

== system mach_lib/claw_main/vel_loops/to full att/e cmd ==
  d_cmd : Inport
  cam : Inport  Port=2
  Demux : Demux  Outputs=[ 2 MACH.num_u_throt ]
  Mux : Mux  Inputs=2
  Mux1 : Mux  Inputs=2
  Mux4 : Mux  Inputs=2
  att2e : utility_lib/att2e  quat_IC=MACH_quat_IC
  att,T : Outport
  e,T : Outport  Port=2
  wires:
  Mux1/1 -> e,T/1
  att2e/1 -> Mux1/1
  Mux/1 -> att,T/1
  d_cmd/1 -> Demux/1
  Mux4/1 -> att2e/1, Mux/1  "att"
  cam/1 -> Mux4/2
  Demux/1 -> Mux4/1
  Demux/2 -> Mux1/2, Mux/2  "throt"

== system mach_lib/claw_main/vel_loops/xu2d ==
  X : Inport
  U : Inport  Port=2
  params : Inport  Port=3
  Assignment : Assignment  Elements=MACH.throttle_idx  OutputInitialize=Initialize using input (U1)
  Bus Selector : BusSelector  OutputSignals=u_llim,u_ulim
  Demux : Demux  Outputs=[ 2 1 ]
  MinMax : MinMax  Inputs=2  SaturateOnIntegerOverflow=on  InputSameDT=on
  MinMax1 : MinMax  Function=max  Inputs=2  SaturateOnIntegerOverflow=on  InputSameDT=on
  Mux : Mux  Inputs=2
  Reshape : simulink/Math Operations/Reshape  OutputDimensionality=1-D array  OutputDimensions=[1,1]
  Selector1 : Selector  Elements=MACH.quat_idx  InputPortWidth=MACH.num_x
  Selector2 : Selector  Elements=MACH.throttle_idx  InputPortWidth=MACH.num_u
  Selector3 : Selector  Elements=3:MACH.vel_num_u  InputPortWidth=MACH.vel_num_u
  Selector4 : Selector  Elements=3:MACH.vel_num_u  InputPortWidth=MACH.vel_num_u
  e2att : utility_lib/e2att
  U_limited : Outport
  d_nom : Outport  Port=2
  cam : Outport  Port=3
  wires:
  Reshape/1 -> Mux/2
  e2att/1 -> Demux/1
  Assignment/1 -> U_limited/1
  MinMax/1 -> Reshape/1, Assignment/2
  Selector3/1 -> MinMax1/2
  Selector4/1 -> MinMax/2
  Bus Selector/2 -> Selector4/1  "<u_ulim>"
  MinMax1/1 -> MinMax/1
  Bus Selector/1 -> Selector3/1  "<u_llim>"
  params/1 -> Bus Selector/1
  Demux/2 -> cam/1
  Demux/1 -> Mux/1
  U/1 -> Assignment/1, Selector2/1
  X/1 -> Selector1/1
  Mux/1 -> d_nom/1
  Selector2/1 -> MinMax1/1  "throttle"
  Selector1/1 -> e2att/1

== system mach_lib/control input/form control input/add effector control params ==
  full_surf_cmd : Inport
  Bus Creator : BusCreator  Inputs=9
  From Workspace : FromWorkspace  VariableName=full_surf_limits_fw.obac.ulim  SampleTime=MACH.dt  Interpolate=off  OutputAfterFinalValue=Holding final value
  From Workspace1 : FromWorkspace  VariableName=full_surf_limits_fw.obac.llim  SampleTime=MACH.dt  Interpolate=off  OutputAfterFinalValue=Holding final value
  From Workspace2 : FromWorkspace  VariableName=full_surf_limits_fw.obac.limit_select  SampleTime=MACH.dt  Interpolate=off  OutputAfterFinalValue=Holding final value
  From Workspace3 : FromWorkspace  VariableName=full_surf_limits_fw.obac.urlim  SampleTime=MACH.dt  Interpolate=off  OutputAfterFinalValue=Holding final value
  From Workspace4 : FromWorkspace  VariableName=full_surf_limits_fw.obac.lrlim  SampleTime=MACH.dt  Interpolate=off  OutputAfterFinalValue=Holding final value
  From Workspace5 : FromWorkspace  VariableName=full_surf_limits_fw.obac.pref_select  SampleTime=MACH.dt  Interpolate=off  OutputAfterFinalValue=Holding final value
  From Workspace6 : FromWorkspace  VariableName=full_surf_limits_fw.obac.pref  SampleTime=MACH.dt  Interpolate=off  OutputAfterFinalValue=Holding final value
  From Workspace7 : FromWorkspace  VariableName=full_surf_limits_fw.obac.pref_wght  SampleTime=MACH.dt  Interpolate=off  OutputAfterFinalValue=Holding final value
  full_surf : Outport
  wires:
  From Workspace1/1 -> Bus Creator/3  "full_surf_llim"
  From Workspace/1 -> Bus Creator/2  "full_surf_ulim"
  full_surf_cmd/1 -> Bus Creator/1  "full_surf_cmd"
  Bus Creator/1 -> full_surf/1
  From Workspace3/1 -> Bus Creator/4  "full_surf_urlim"
  From Workspace4/1 -> Bus Creator/5  "full_surf_lrlim"
  From Workspace2/1 -> Bus Creator/6  "full_surf_lock"
  From Workspace5/1 -> Bus Creator/7  "full_surf_pref_select"
  From Workspace6/1 -> Bus Creator/8  "full_surf_pref"
  From Workspace7/1 -> Bus Creator/9  "full_surf_pref_wght"

== system mach_lib/control input/form control input/engine parameters ==
  Bus Creator2 : BusCreator  Inputs=3
  Constant : Constant  Value=obac_params.Isp_sl
  Constant1 : Constant  Value=obac_params.Isp_vacuum
  Constant2 : Constant  Value=obac_params.throt_to_ff
  engines : Outport
  wires:
  Constant1/1 -> Bus Creator2/2  "Isp_vacuum"
  Constant/1 -> Bus Creator2/1  "Isp_sl"
  Bus Creator2/1 -> engines/1
  Constant2/1 -> Bus Creator2/3  "throt_to_ff"

== system mach_lib/control input/form control input/mode switches ==
  control_input : Inport
  Bus Creator1 : BusCreator  Inputs=17
  Bus Selector4 : BusSelector  OutputSignals=CLAW_mode,accel_submode
  Compare To Zero : simulink/Logic and Bit Operations/Compare To Zero  relop=>  LogicOutDataTypeMode=boolean  ZeroCross=off
  Data Type Conversion : DataTypeConversion
  From Workspace : FromWorkspace  VariableName=enable_bb_fw  SampleTime=MACH.dt  Interpolate=off  OutputAfterFinalValue=Holding final value
  From Workspace1 : FromWorkspace  VariableName=use_att_rate_cmd_fw  SampleTime=MACH.dt  Interpolate=off  OutputAfterFinalValue=Holding final value
  From Workspace2 : FromWorkspace  VariableName=use_cam_rate_cmd_fw  SampleTime=MACH.dt  Interpolate=off  OutputAfterFinalValue=Holding final value
  From Workspace3 : FromWorkspace  VariableName=enable_homing_fw  SampleTime=MACH.dt  Interpolate=off  OutputAfterFinalValue=Holding final value
  From Workspace4 : FromWorkspace  VariableName=nav_enable_fw  SampleTime=MACH.dt  Interpolate=off  OutputAfterFinalValue=Holding final value
  From Workspace5 : FromWorkspace  VariableName=gain_set_fw  SampleTime=MACH.dt  Interpolate=off  OutputAfterFinalValue=Holding final value
  From Workspace6 : FromWorkspace  VariableName=att_type_fw  SampleTime=MACH.dt  Interpolate=off  OutputAfterFinalValue=Holding final value
  From Workspace7 : FromWorkspace  VariableName=use_held_aero_obac_fw  SampleTime=MACH.dt  Interpolate=off  OutputAfterFinalValue=Holding final value
  int_reset_sw : Constant  Value=0
  llh_input_sw : Constant  Value=0
  pre_takeoff_sw : Constant  Value=0
  reset_pos_sw : Constant  Value=0
  use_full_surf_cmd_sw : Constant  Value=use_full_surf_cmd
  wind_est_sw : Constant  Value=0
  mode_sw : Outport
  wires:
  reset_pos_sw/1 -> Bus Creator1/5  "reset_pos_sw"
  wind_est_sw/1 -> Bus Creator1/6  "wind_est_sw"
  llh_input_sw/1 -> Bus Creator1/7  "llh_input_sw"
  Compare To Zero/1 -> Data Type Conversion/1  "engaged_sw"
  pre_takeoff_sw/1 -> Bus Creator1/4  "pre_takeoff_sw"
  int_reset_sw/1 -> Bus Creator1/8  "int_reset_sw"
  Data Type Conversion/1 -> Bus Creator1/2  "engaged_sw"
  use_full_surf_cmd_sw/1 -> Bus Creator1/11  "full_surf_cmd_sw"
  From Workspace2/1 -> Bus Creator1/10  "cam_rate_cmd_sw"
  From Workspace6/1 -> Bus Creator1/9  "att_type"
  From Workspace3/1 -> Bus Creator1/12  "enable_homing_sw"
  From Workspace1/1 -> Bus Creator1/13  "att_rate_cmd_sw"
  From Workspace4/1 -> Bus Creator1/14  "nav_enable_sw"
  From Workspace/1 -> Bus Creator1/15  "enable_bb_sw"
  From Workspace5/1 -> Bus Creator1/16  "gain_set_sw"
  From Workspace7/1 -> Bus Creator1/17  "use_held_aero_obac_sw"
  Bus Selector4/2 -> Bus Creator1/3  "<accel_submode>"
  Bus Creator1/1 -> mode_sw/1
  control_input/1 -> Bus Selector4/1
  Bus Selector4/1 -> Compare To Zero/1, Bus Creator1/1  "<CLAW_mode>"

== system mach_lib/control input/form control input/select command ==
  cmd_bus : Inport
  Bus Creator1 : BusCreator
  Bus Selector : BusSelector  OutputSignals=da_cmd,de_cmd,dr_cmd,throttle_cmd  OutputAsBus=on
  Bus Selector4 : BusSelector  OutputSignals=full_surf_cmd,accel_submode,CLAW_mode
  Multiport Switch : MultiPortSwitch  Inputs=5  zeroidx=on  SaturateOnIntegerOverflow=on
  att cmd select : Subsystem
  pos cmd select : Subsystem
  rate cmd select : Subsystem
  vel cmd select : Subsystem
  control_input : Outport
  wires:
  Multiport Switch/1 -> Bus Creator1/4  "command"
  pos cmd select/1(pos_cmd) -> Multiport Switch/6
  att cmd select/1(att_cmd) -> Multiport Switch/4
  rate cmd select/1(rate_cmd) -> Multiport Switch/3
  Bus Selector/1 -> Multiport Switch/2
  Bus Selector4/3 -> Multiport Switch/1, Bus Creator1/3  "<CLAW_mode>"
  cmd_bus/1 -> pos cmd select/1(cmd_bus), vel cmd select/1(cmd_bus), Bus Selector4/1, Bus Selector/1, rate cmd select/1(cmd_bus), att cmd select/1(cmd_bus)
  vel cmd select/1(vel_cmd) -> Multiport Switch/5
  Bus Selector4/2 -> Bus Creator1/2  "<accel_submode>"
  Bus Selector4/1 -> Bus Creator1/1  "<full_surf_cmd>"
  Bus Creator1/1 -> control_input/1

== system mach_lib/control input/generate commands/pos cmd generator ==
  cmd_bus : Inport
  From Workspace5 : FromWorkspace  VariableName=pos_cmd_fw  SampleTime=MACH.dt  OutputAfterFinalValue=Holding final value
  Ground : Ground
  Multiport Switch2 : MultiPortSwitch  zeroidx=on  SaturateOnIntegerOverflow=on
  circle pos cmd : Subsystem
  ramp pos cmd : Subsystem
  use_cam_rate_cmd1 : Constant  Value=pos_cmd_select
  pos_cmd : Outport
  wires:
  Ground/1 -> Multiport Switch2/2
  From Workspace5/1 -> Multiport Switch2/3
  use_cam_rate_cmd1/1 -> Multiport Switch2/1
  Multiport Switch2/1 -> pos_cmd/1
  ramp pos cmd/1(pos_cmd) -> Multiport Switch2/4
  circle pos cmd/1(pos_cmd) -> Multiport Switch2/5
  cmd_bus/1 -> ramp pos cmd/1(cmd_bus), circle pos cmd/1(cmd_bus)

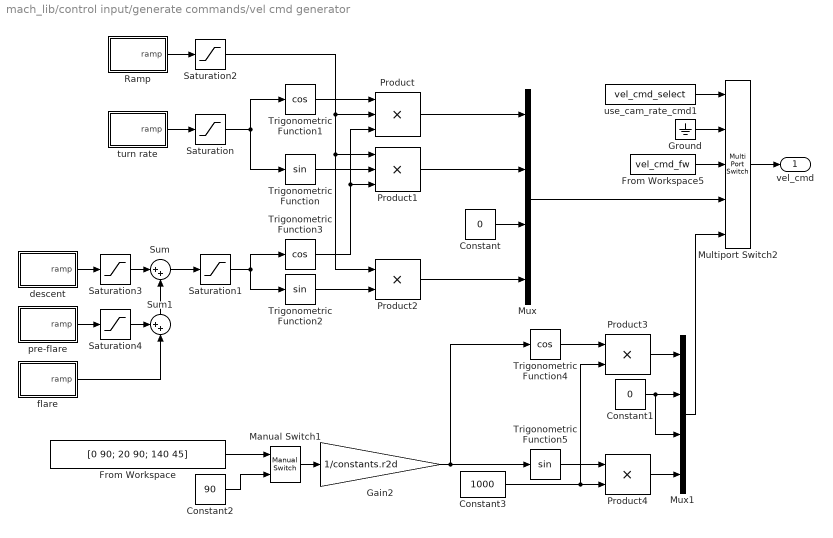
== system mach_lib/control input/generate commands/vel cmd generator ==
  Constant : Constant  Value=0
  Constant1 : Constant  Value=0
  Constant2 : Constant  Value=90
  Constant3 : Constant  Value=1000
  From Workspace : FromWorkspace  VariableName=[0 90; 20 90; 140 45]  SampleTime=MACH.dt  OutputAfterFinalValue=Holding final value
  From Workspace5 : FromWorkspace  VariableName=vel_cmd_fw  SampleTime=MACH.dt  OutputAfterFinalValue=Holding final value
  Gain2 : Gain  Gain=1/constants.r2d
  Ground : Ground
  Manual Switch1 : simulink/Signal Routing/Manual Switch  sw=1  action=0
  Multiport Switch2 : MultiPortSwitch  zeroidx=on  SaturateOnIntegerOverflow=on
  Mux : Mux
  Mux1 : Mux
  Product : Product  Inputs=3  SaturateOnIntegerOverflow=on
  Product1 : Product  Inputs=3  SaturateOnIntegerOverflow=on
  Product2 : Product  SaturateOnIntegerOverflow=on
  Product3 : Product  SaturateOnIntegerOverflow=on
  Product4 : Product  SaturateOnIntegerOverflow=on
  Ramp : Subsystem  mask{slope=accel_cmd, start_time=time_accel_cmd, initial_output=Nd_trim_IC, sample_time=MACH.dt}
      mask prompts: start_time "Start time:"; initial_output "Initial output:"; sample_time "Sample time (-1 for inherited):"
  Saturation : Saturate  UpperLimit=max_chi_cmd  LowerLimit=min_chi_cmd
  Saturation1 : Saturate  UpperLimit=0  LowerLimit=gam_cmd_descent
  Saturation2 : Saturate  UpperLimit=max_vel_cmd  LowerLimit=min_vel_cmd
  Saturation3 : Saturate  UpperLimit=0  LowerLimit=gam_cmd_descent
  Saturation4 : Saturate  UpperLimit=-gam_cmd_descent + gam_cmd_preflare  LowerLimit=-inf
  Sum : Sum  Inputs=|++
  Sum1 : Sum  Orientation=up  Inputs=++|
  Trigonometric Function : Trigonometry
  Trigonometric Function1 : Trigonometry  Operator=cos
  Trigonometric Function2 : Trigonometry
  Trigonometric Function3 : Trigonometry  Operator=cos
  Trigonometric Function4 : Trigonometry  Operator=cos
  Trigonometric Function5 : Trigonometry
  descent : Subsystem  mask{slope=gamdot_cmd_descent, start_time=time_gamdot_cmd_descent, initial_output=0, sample_time=MACH.dt}
      mask prompts: start_time "Start time:"; initial_output "Initial output:"; sample_time "Sample time (-1 for inherited):"
  flare : Subsystem  mask{slope=gamdot_cmd_flare, start_time=time_gamdot_cmd_flare, initial_output=0, sample_time=MACH.dt}
      mask prompts: start_time "Start time:"; initial_output "Initial output:"; sample_time "Sample time (-1 for inherited):"
  pre-flare : Subsystem  mask{slope=gamdot_cmd_preflare, start_time=time_gamdot_cmd_preflare, initial_output=0, sample_time=MACH.dt}
      mask prompts: start_time "Start time:"; initial_output "Initial output:"; sample_time "Sample time (-1 for inherited):"
  turn rate : Subsystem  mask{slope=turn_rate_cmd, start_time=time_turn_cmd, initial_output=0, sample_time=MACH.dt}
      mask prompts: start_time "Start time:"; initial_output "Initial output:"; sample_time "Sample time (-1 for inherited):"
  use_cam_rate_cmd1 : Constant  Value=vel_cmd_select
  vel_cmd : Outport
  wires:
  Trigonometric Function1/1 -> Product/1
  Trigonometric Function/1 -> Product1/2
  turn rate/1(ramp) -> Saturation/1
  Saturation/1 -> Trigonometric Function1/1, Trigonometric Function/1
  Product/1 -> Mux/1
  Product1/1 -> Mux/2
  Ramp/1(ramp) -> Saturation2/1
  Saturation1/1 -> Trigonometric Function3/1, Trigonometric Function2/1
  Trigonometric Function3/1 -> Product/3, Product1/3
  Product2/1 -> Mux/4
  Trigonometric Function2/1 -> Product2/2
  Saturation2/1 -> Product/2, Product1/1, Product2/1
  descent/1(ramp) -> Saturation3/1
  Sum/1 -> Saturation1/1
  Saturation3/1 -> Sum/1
  Constant/1 -> Mux/3
  pre-flare/1(ramp) -> Saturation4/1
  Sum1/1 -> Sum/2
  flare/1(ramp) -> Sum1/2
  Saturation4/1 -> Sum1/1
  Multiport Switch2/1 -> vel_cmd/1
  Constant1/1 -> Mux1/2, Mux1/3
  Trigonometric Function4/1 -> Product3/1
  Product3/1 -> Mux1/1
  Trigonometric Function5/1 -> Product4/1
  Product4/1 -> Mux1/4
  Mux1/1 -> Multiport Switch2/5
  Gain2/1 -> Trigonometric Function4/1, Trigonometric Function5/1
  Manual Switch1/1 -> Gain2/1
  From Workspace/1 -> Manual Switch1/1
  Constant2/1 -> Manual Switch1/2
  Mux/1 -> Multiport Switch2/4
  use_cam_rate_cmd1/1 -> Multiport Switch2/1
  From Workspace5/1 -> Multiport Switch2/3
  Constant3/1 -> Product4/2, Product3/2
  Ground/1 -> Multiport Switch2/2

== system mach_lib/sim params/winds/wind dblt ==
  Constant : Constant  Value=wind_omega
  Constant1 : Constant  Orientation=down
  Gain : Gain  Gain=0.5*wind2  SaturateOnIntegerOverflow=on
  Nwind Step : Step  Time=5  After=wind1  SampleTime=dtsim
  Product : Product  SaturateOnIntegerOverflow=on
  Product1 : Product  Inputs=3  SaturateOnIntegerOverflow=on
  Rate Limiter : RateLimiter  RisingSlewLimit=5  FallingSlewLimit=-5
  Sum1 : Sum  Inputs=+-|  SaturateOnIntegerOverflow=on
  Sum5 : Sum  Inputs=|++  SaturateOnIntegerOverflow=on
  Trigonometric Function : Trigonometry  Operator=cos
  change sign : Step  Time=wind_pulse_time + 2 * pi / wind_omega  Before=1  After=-1  SampleTime=dtsim
  time : simulink/Sources/Ramp  slope=1  start=wind_pulse_time  X0=0
  turn off : Step  Time=wind_pulse_time + 4 * pi / wind_omega  Before=1  After=0  SampleTime=0
  Out1 : Outport
  wires:
  change sign/1 -> Product1/3
  Nwind Step/1 -> Rate Limiter/1
  Rate Limiter/1 -> Sum5/2
  Sum5/1 -> Out1/1
  Gain/1 -> Sum5/1
  Product1/1 -> Gain/1
  turn off/1 -> Product1/2
  Sum1/1 -> Product1/1
  Constant1/1 -> Sum1/1
  Trigonometric Function/1 -> Sum1/2
  Product/1 -> Trigonometric Function/1
  Constant/1 -> Product/2
  time/1 -> Product/1

== system mach_lib/sim params/winds/wind pulse ==
  Constant : Constant  Value=wind_omega
  Constant1 : Constant  Orientation=down
  Gain : Gain  Gain=0.5*wind2  SaturateOnIntegerOverflow=on
  Nwind Step : Step  Time=5  After=wind1  SampleTime=dtsim
  Product : Product  SaturateOnIntegerOverflow=on
  Product1 : Product  SaturateOnIntegerOverflow=on
  Rate Limiter : RateLimiter  RisingSlewLimit=0.5  FallingSlewLimit=-0.5
  Sum1 : Sum  Inputs=+-|  SaturateOnIntegerOverflow=on
  Sum5 : Sum  Inputs=|++  SaturateOnIntegerOverflow=on
  Trigonometric Function : Trigonometry  Operator=cos
  time : simulink/Sources/Ramp  slope=1  start=wind_pulse_time  X0=0
  turn off : Step  Time=wind_pulse_time + 2 * pi / wind_omega  Before=1  After=0  SampleTime=dtsim
  Out1 : Outport
  wires:
  Nwind Step/1 -> Rate Limiter/1
  Rate Limiter/1 -> Sum5/2
  Sum5/1 -> Out1/1
  Gain/1 -> Sum5/1
  Product1/1 -> Gain/1
  turn off/1 -> Product1/2
  Sum1/1 -> Product1/1
  Constant1/1 -> Sum1/1
  Trigonometric Function/1 -> Sum1/2
  Product/1 -> Trigonometric Function/1
  Constant/1 -> Product/2
  time/1 -> Product/1

== system mach_lib/sim params/winds/wind shear ==
  Nwind Step : Step  Orientation=left  Time=5  After=wind1  SampleTime=dtsim
  Nwind shear : simulink/Sources/Ramp  Orientation=left  slope=wind3  start=90  X0=0
  Rate Limiter : RateLimiter  Orientation=left  RisingSlewLimit=0.25  FallingSlewLimit=-0.25
  Saturation2 : Saturate  Orientation=left  UpperLimit=abs(wind2)  LowerLimit=-abs(wind2)
  Sum5 : Sum  Orientation=left  Inputs=++|  SaturateOnIntegerOverflow=on
  Out1 : Outport  Orientation=left
  wires:
  Sum5/1 -> Out1/1
  Rate Limiter/1 -> Sum5/1
  Nwind Step/1 -> Rate Limiter/1
  Saturation2/1 -> Sum5/2
  Nwind shear/1 -> Saturation2/1

== system mach_lib/claw_main/att_loops/dyn inv/Limit rate cmd ==
  limit_pqr_cmd : Inport
  uvw : Inport  Port=2
  pqr : Inport  Port=3
  Constant1 : Constant  Value=MACH.az_llim
  Constant2 : Constant  Value=MACH.att_u_llim
  Constant3 : Constant  Value=MACH.att_u_ulim
  Constant4 : Constant  Value=MACH.az_ulim
  Enforce lower limit : MinMax  Function=max  Inputs=2  OutScaling=2^-10  ZeroCross=off
  Enforce upper limit : MinMax  Inputs=2  OutScaling=2^-10  ZeroCross=off
  Multiport Switch : MultiPortSwitch  Inputs=2  zeroidx=on
  velocity based angular rate llim : mach_lib/velocity based angular rate limit  q_idx=2
  velocity based angular rate ulim : mach_lib/velocity based angular rate limit  q_idx=2
  pqr_limited : Outport
  wires:
  limit_pqr_cmd/1 -> Multiport Switch/1
  Multiport Switch/1 -> pqr_limited/1
  Enforce upper limit/1 -> Multiport Switch/3
  velocity based angular rate llim/1 -> Enforce lower limit/2
  Constant3/1 -> velocity based angular rate ulim/1  "upper_limit"
  Constant1/1 -> velocity based angular rate ulim/2
  Constant4/1 -> velocity based angular rate llim/2
  Constant2/1 -> velocity based angular rate llim/1
  uvw/1 -> velocity based angular rate llim/3, velocity based angular rate ulim/3
  velocity based angular rate ulim/1 -> Enforce upper limit/2
  pqr/1 -> Multiport Switch/2, Enforce lower limit/1
  Enforce lower limit/1 -> Enforce upper limit/1

== system mach_lib/claw_main/att_loops/select att cmd/get direct cmd ==
  signal_bus : Inport
  Bus Selector : BusSelector  OutputSignals=cmd_bus.autopilot_cmd,mode_sw.full_surf_cmd_sw,full_surf.full_surf_cmd
  Demux1 : Demux  Outputs=[ 3 1 ]
  Gain : Gain  Gain=MACH.throt_mixer
  Multiport Switch2 : MultiPortSwitch  Inputs=2  zeroidx=on
  throttle : Selector  Elements=MACH.throttle_idx  InputPortWidth=MACH.num_u
  att : Outport
  throt : Outport  Port=2
  wires:
  Multiport Switch2/1 -> throt/1
  throttle/1 -> Multiport Switch2/3
  Bus Selector/3 -> throttle/1  "<full_surf_cmd>"
  Gain/1 -> Multiport Switch2/2
  Bus Selector/2 -> Multiport Switch2/1  "<full_surf_cmd_sw>"
  Bus Selector/1 -> Demux1/1  "<autopilot_cmd>"
  signal_bus/1 -> Bus Selector/1
  Demux1/2 -> Gain/1
  Demux1/1 -> att/1
